simulink model "Battery_SC_NTSMC_NN"  (R2021a)
settings: Solver=ode23tb  StartTime=0.0  StopTime=5  MaxStep=1e-4  RelTol=1e-3
values from neighbouring files (symbols this model uses):
  C = 1e-12    [MPPTNN.m]    (also in NN_Tph.m)
  L = 100e-3    (= 0.1)    [MPPTNN.m]    (also in NN_Tph.m)
  Lf = 10e-3    (= 0.01)    [MPPTNN.m]    (also in NN_Tph.m)
  Ll = 31e-6    (= 3.1e-05)    [MPPTNN.m]    (also in NN_Tph.m)
  R = 4.33    [MPPTNN.m]    (also in NN_Tph.m)
  Rf = 40e-3    (= 0.04)    [MPPTNN.m]    (also in NN_Tph.m)
  RL = 0.1    [MPPTNN.m]    (also in NN_Tph.m)
  Ts = 0.50e-5    (= 5e-06)    [MPPTNN.m]    (also in NN_Tph.m)
undefined symbols (not defined in the file or in its folder): Ion, Lithium, sigbuilder_block
libraries: neural x125, spsFirstOrderFilterLib x11, spsSeriesRLCBranchLib x10, spsIGBTDiodeLib x5, spsPWMGeneratorDCDCLib x5, simulink x5, spsMeanLib x5, pid_lib x4, spsDiodeLib x4, spsabctodq0Lib x3, spsThreePhaseSeriesRLCBranchLib x2, spsRMSLib x2
(part 1 of 4)
settings Model: Creator=Rodayna  LastModifiedBy=Morteza Pirmohammad
settings SolverCC: AlgebraicLoopSolver=TrustRegion
settings DataIOCC: ReturnWorkspaceOutputs=off
settings DebuggingCC: SFMachineParentedDataDiag=warning  ArithmeticOperatorsInVariantConditions=warning
settings SFSimCC: SimUseLocalCustomCode=off  CustomCodeUndefinedFunction=UseInterfaceOnly
settings RTWCC: RTWUseLocalCustomCode=off
settings CodeAppCC: StateflowObjectComments=on
settings SimscapeCC: SimscapeNormalizeSystem=off

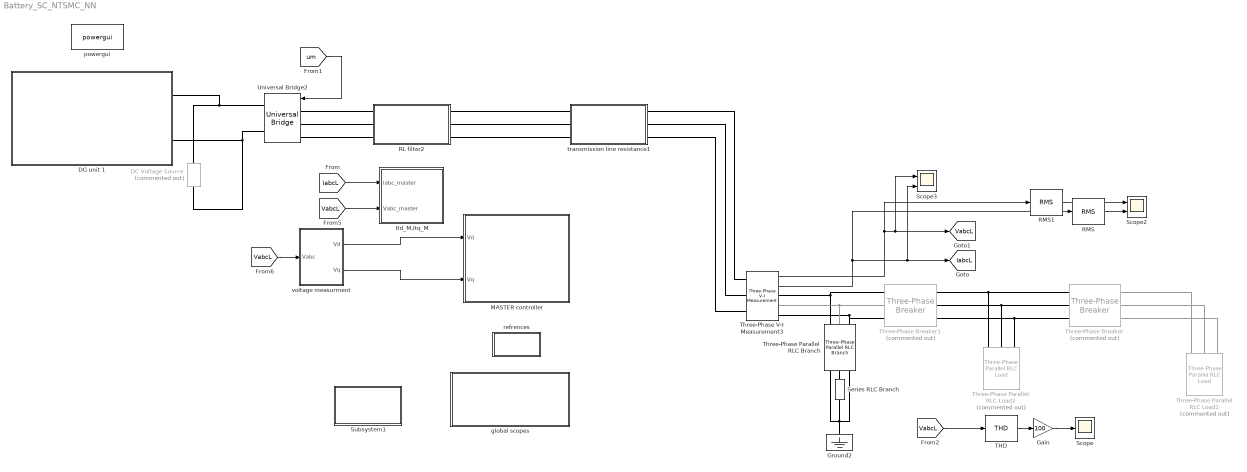
== system Battery_SC_NTSMC_NN ==
  DC Voltage Source : spsDCVoltageSourceLib/DC Voltage Source  Commented=on  Amplitude=100  Measurements=None
  DG unit 1 : Subsystem
  Gain : Gain  Gain=100
  Ground2 : spsGroundLib/Ground  LConnTagsString=a
  Itd_M,Itq_M : Subsystem
  MASTER controller : Subsystem
  RL filter2 : Subsystem
  RMS : spsRMSLib/RMS  TrueRMS=on  Freq=50  RMSInit=0  Ts=0
  RMS1 : spsRMSLib/RMS  TrueRMS=on  Freq=50  RMSInit=0  Ts=0
  Scope : Scope
  Scope2 : Scope  NumInputPorts=2
  Scope3 : Scope  NumInputPorts=2
  Series RLC Branch : spsSeriesRLCBranchLib/Series RLC Branch  LConnTagsString=__new0  RConnTagsString=__new0  BranchType=R  Resistance=0.1  Inductance=1e-3  SetiL0=off  InitialCurrent=0  Capacitance=1e-6  Setx0=off  InitialVoltage=0  Measurements=None
  Subsystem1 : Subsystem
  THD : spsTHDLib/THD  Freq=50  Ts=0
      settings: SourceProductBaseCode=PS
  Three-Phase Parallel RLC Branch : spsThreePhaseParallelRLCBranchLib/Three-Phase Parallel RLC Branch  LConnTagsString=A|B|C  RConnTagsString=A|B|C  BranchType=RLC  Resistance=R  Inductance=L  Capacitance=C  Measurements=Branch voltages and currents
      settings: SourceProductBaseCode=PS
  Three-Phase Parallel RLC Load1 : spsThreePhaseParallelRLCLoadLib/Three-Phase Parallel RLC Load  Commented=on  LConnTagsString=A|B|C  Configuration=Y (grounded)  NominalVoltage=380  Vabc=[1e3 1e3 1e3]  Vabcp=[1e3 1e3 1e3]  NominalFrequency=50  UnbalancedPower=off  ActivePower=5e3  InductivePower=0  CapacitivePower=0  Pabc=[10e3 9e3 11e3]  QLabc=[100 90 110]  QCabc=[100 90 110]  Pabcp=[10e3 9e3 11e3]  QLabcp=[100 90 110]  QCabcp=[100 90 110]  Measurements=None  LoadType=constant Z
  Three-Phase Parallel RLC Load2 : spsThreePhaseParallelRLCLoadLib/Three-Phase Parallel RLC Load  Commented=on  LConnTagsString=A|B|C  Configuration=Y (grounded)  NominalVoltage=380  Vabc=[1e3 1e3 1e3]  Vabcp=[1e3 1e3 1e3]  NominalFrequency=50  UnbalancedPower=off  ActivePower=10e3  InductivePower=5e3  CapacitivePower=0  Pabc=[10e3 9e3 11e3]  QLabc=[100 90 110]  QCabc=[100 90 110]  Pabcp=[10e3 9e3 11e3]  QLabcp=[100 90 110]  QCabcp=[100 90 110]  Measurements=None  LoadType=constant PQ
  Three-Phase V-I Measurement3 : spsThreePhaseVIMeasurementLib/Three-Phase V-I Measurement  VoltageMeasurement=phase-to-ground  SetLabelV=off  LabelV=Vabc  Vpu=off  VpuLL=off  CurrentMeasurement=yes  SetLabelI=off  LabelI=Iabc  Ipu=off  Pbase=100e6  Vbase=500e3  OutputType=Complex  PhasorSimulation=off  PSBequivalent=0
  Three-Phase Breaker : spsThreePhaseBreakerLib/Three-Phase Breaker  Commented=on  InitialState=open  SwitchA=on  SwitchB=on  SwitchC=on  SwitchTimes="[2  3]"  External=off  BreakerResistance=0.01  SnubberResistance=1e6  SnubberCapacitance=inf  Measurements=None
  Three-Phase Breaker1 : spsThreePhaseBreakerLib/Three-Phase Breaker  Commented=on  InitialState=open  SwitchA=on  SwitchB=on  SwitchC=on  SwitchTimes="[1  4]"  External=off  BreakerResistance=0.01  SnubberResistance=1e6  SnubberCapacitance=inf  Measurements=None
  Universal Bridge2 : spsUniversalBridgeLib/Universal Bridge  Arms=3  SnubberResistance=1e3  SnubberCapacitance=inf  Device=MOSFET / Diodes  Ron=1e-3  Lon=0  ForwardVoltages="[  0  0  ]"  ForwardVoltage=0  GTOparameters=[ 10e-6 , 20e-6 ]  IGBTparameters=[ 1e-6 , 2e-6 ]  Measurements=None  Measurements_2=None  converterType=Rectifier
  global scopes : Subsystem
  powergui : spspowerguiLib/powergui  Priority=1  SimulationMode=Discrete  SampleTime=Ts  frequency=60  Iterations=50  frequencyindice=0  Pbase=100e6  ErrMax=1e-4  UnitsV=kV  UnitsW=MW  buscounter=0  FunctionMessages=off  echomessages=off  EnableUseOfTLC=off  CurrentSourceSwitches=off  DisableSnubberDevices=off  DisableRonSwitches=off  DisableVfSwitches=off  DisplayEquations=off  AutomaticDiscreteSolvers=off  SolverType=Tustin/Backward Euler (TBE)  Interpol=off  ExternalGateDelay=off  methode=off  Ts=100  x0status=blocks  SPID=on  SwTol=0  HookPort=off  NonlinearTolerance=1e-4  nMaxIteration=100  ContinueOnMaxIteration=off  RestoreLinks=warning  ResistiveCurrentMeasurement=off  Frange=[0:2:500]  Ylog=off  Xlog=on  ShowGrid=off  save=off  variable=ZData  structure=0  ZoomFFT=off  StartTime=0.0  cycles=1  DisplayStyle=1  fundamental=60  FreqAxis=off  MaxFrequency=1000  frequencyindicesteady=1  RmsSteady=1  display=off
  refrences : Subsystem
  transmission line resistance1 : Subsystem
  voltage measurment : Subsystem
  tag scope: IabcL=global, VabcL=global
  wires:
  voltage measurment/2(Vq) -> MASTER controller/2(Vq)
  voltage measurment/1(Vd) -> MASTER controller/1(Vd)
  [VabcL] -> Itd_M,Itq_M/2(Vabc_master)
  [VabcL] -> voltage measurment/1(Vabc)
  [IabcL] -> Itd_M,Itq_M/1(Iabc_master)
  [um] -> Universal Bridge2/1
  RMS/1 -> Scope2/2
  RMS1/1 -> Scope2/1
  Three-Phase V-I Measurement3/1 -> RMS1/1, Scope3/1, [VabcL]
  Three-Phase V-I Measurement3/2 -> RMS/1, Scope3/2, [IabcL]
  Gain/1 -> Scope/1
  THD/1 -> Gain/1
  [VabcL] -> THD/1
  connections:
  DG unit 1/RConn1 -- Universal Bridge2/RConn1 -- DC Voltage Source/RConn1
  DG unit 1/RConn2 -- DC Voltage Source/LConn1 -- Universal Bridge2/RConn2
  transmission line resistance1/LConn3 -- RL filter2/RConn3
  transmission line resistance1/LConn1 -- RL filter2/RConn1
  RL filter2/RConn2 -- transmission line resistance1/LConn2
  Universal Bridge2/LConn2 -- RL filter2/LConn2
  Universal Bridge2/LConn1 -- RL filter2/LConn1
  Universal Bridge2/LConn3 -- RL filter2/LConn3
  Three-Phase Parallel RLC Branch/LConn3 -- Three-Phase V-I Measurement3/RConn3 -- Three-Phase Breaker1/LConn3
  Three-Phase Parallel RLC Branch/LConn1 -- Three-Phase V-I Measurement3/RConn1 -- Three-Phase Breaker1/LConn1
  Three-Phase Parallel RLC Load2/LConn2 -- Three-Phase Breaker/LConn2 -- Three-Phase Breaker1/RConn2
  Three-Phase Parallel RLC Branch/RConn1 -- Ground2/LConn1 -- Series RLC Branch/RConn1 -- Three-Phase Parallel RLC Branch/RConn3
  Three-Phase Parallel RLC Load2/LConn1 -- Three-Phase Breaker/LConn1 -- Three-Phase Breaker1/RConn1
  Three-Phase Breaker1/LConn2 -- Three-Phase Parallel RLC Branch/LConn2 -- Three-Phase V-I Measurement3/RConn2
  Three-Phase Parallel RLC Load2/LConn3 -- Three-Phase Breaker/LConn3 -- Three-Phase Breaker1/RConn3
  Series RLC Branch/LConn1 -- Three-Phase Parallel RLC Branch/RConn2
  transmission line resistance1/RConn1 -- Three-Phase V-I Measurement3/LConn1
  Three-Phase Breaker/RConn2 -- Three-Phase Parallel RLC Load1/LConn2
  Three-Phase Breaker/RConn3 -- Three-Phase Parallel RLC Load1/LConn3
  Three-Phase V-I Measurement3/LConn2 -- transmission line resistance1/RConn2
  Three-Phase V-I Measurement3/LConn3 -- transmission line resistance1/RConn3
  Three-Phase Breaker/RConn1 -- Three-Phase Parallel RLC Load1/LConn1

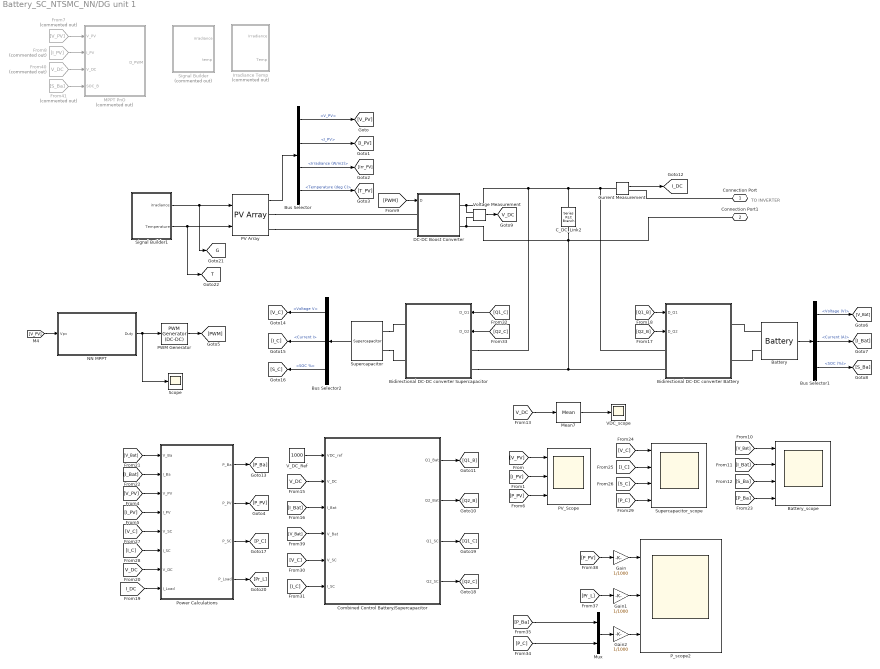
== system Battery_SC_NTSMC_NN/DG unit 1 ==
  note: TO INVERTER
  Battery : spsBatteryLib/Battery  BatType=Lithium-Ion  ShowTempParam=off  ThermalPreset=no  ShowAgeParam=off  NomV=750  NomQ=40  SOC=50  Batt_Tr=0.1  PresetModel=on  MaxQ=40  MinV=562.5  FullV=872.9904  Dis_rate=17.3913  R=0.1875  Normal_OP=36.1739  expZone="[810.2894      1.965217]"  current=[17.5 35 52]  Units=Time  Tci=20  NomT=20  T2=-30  MaxQ2=4.8  FullV2=7.1  Normal_OP2=5.655  expZone2="[6.58           1]"  Rca=0.6  ti=2000  Dp=0  Neq0=0  Tsim=1e6  Ta1=25  Qeol=5.4*0.9  Reol=0.013333*1.2  Char_age=[2.3478, 3]  Dis_age=[2.3478, 10]  N1=1500  N2=10500  N3=1000  N4=1400  Ta2=45  N5=950
  "Battery_scope " : Scope  NumInputPorts=4
  Bidirectional DC-DC converter Battery : Subsystem
  Bidirectional DC-DC converter Supercapacitor : Subsystem
  Bus Selector : BusSelector  OutputSignals=V_PV,I_PV,Irradiance (W/m2),Temperature (deg C)
  Bus Selector1 : BusSelector  OutputSignals=Voltage (V),Current (A),SOC (%)
  Bus Selector2 : BusSelector  OutputSignals=Voltage V,Current I,SOC %
  C_DC_Link2 : spsSeriesRLCBranchLib/Series RLC Branch  LConnTagsString=__new0  RConnTagsString=__new0  BranchType=C  Resistance=1  Inductance=1e-3  SetiL0=off  InitialCurrent=0  Capacitance=500e-6  Setx0=off  InitialVoltage=0  Measurements=None
  Combined Control Battery/Supercapacitor : Subsystem
  Current Measurement : spsCurrentMeasurementLib/Current Measurement  PhasorSimulation=off  OutputType=Complex  PSBequivalent=0
  DC-DC Boost Converter : Subsystem
  From40 : From  Commented=on  GotoTag=V_DC  TagVisibility=global
  From41 : From  Commented=on  GotoTag=S_Ba
  From7 : From  Commented=on  GotoTag=V_PV
  From8 : From  Commented=on  GotoTag=I_PV
  Gain : Gain  Gain=1/1000
  Gain1 : Gain  Gain=1/1000
  Gain2 : Gain  Gain=1/1000
  Irradiance Temp : Subsystem  Tag=STV Subsys  Commented=on  LoadFcn=sigbuilder_block('load');  StartFcn=sigbuilder_block('start');  StopFcn=sigbuilder_block('stop');  ClipboardFcn=sigbuilder_block('clipboard');  mask(Sigbuilder block){tuvar=[0:10]}
      mask help: Sigbuilder GUI
      mask init:
      | if ~strcmp(get_param(bdroot(gcbh),'SimulationStatus'),'stopped') tuvar = sigbuilder_block('maskInit'); end
      settings: CopyFcn=sigbuilder_block('copy');  DeleteFcn=sigbuilder_block('delete');  ModelCloseFcn=sigbuilder_block('modelClose');  PreSaveFcn=sigbuilder_block('preSave');  PauseFcn=sigbuilder_block('pause')  ContinueFcn=sigbuilder_block('continue')  NameChangeFcn=sigbuilder_block('namechange');  OpenFcn=sigbuilder_block('open',[6 0 1012.5 477.75 ]);  CloseFcn=sigbuilder_block('close');
      mask Display: plot(0, 0, 100, 100,[2, 2, 32, 32, 2], [68, 8, 8, 68, 68],[32, 2], [38, 38], [32, 19, 2],[53, 60, 44], [32, 17, 17, 2],[16, 16, 31, 31]);txt = getActiveGroup(gcbh);text(2, 100, txt,'verticalAlignment', 'top');
  MPPT PnO : Subsystem  Commented=on
  Mean7 : spsMeanLib/Mean  Freq=60  Vinit=0  Ts=0
  Mux : Mux  Inputs=2
  NN MPPT : Subsystem
      mask help: Custom Neural Network
      mask Display: e = 0.06;c1 = [120 150 230]/255;c2 = ([120 150 230]+0)/383;c3 = ([120 150 230]+128)/383;patch([0 1 1 0],[0 0 1 1],c1);patch([0 1 1 1-e 1-e 0+e],[0 0 1 1-e 0+e 0+e],c2);patch([0 0 1 1-e 0+e 0+e],[0 1 1 1-e 1-e 0+e],c3);plot([0 1 1 0 0],[0 0 1 1 0]);fprintf('NNET');port_label('input',1,' Input');port_label('output',1,'Output ');
  PV Array : spsPVArrayLib/PV Array  Npar=6  Nser=30  PlotType=array @ 25 deg.C & specified irradiances  S_vec="[ 1000 800 500  250 ]"  Temp_C_vec="[0 25 50  ]"  ModuleName=Yingli Energy (China) YL250P-29b  PlotWhenSelected=on  Pm=250.496  Ncell=60  Voc=38.4  Isc=8.79  Vm=30.4  Im=8.24  beta_Voc_pc=-0.337  alpha_Isc_pc=0.0438  beta_Voc=-0.12941  alpha_Isc=0.00385  IL=8.8005  I0=1.272e-10  nI=0.99849  Rsh=362.5163  Rs=0.42475  RobustModel=off  RobustCellTemperature=313.3991  BAL=on  Tc=Tc  Tfilter=5e-5
  PV_Scope : Scope  NumInputPorts=3
  "PWM Generator " : spsPWMGeneratorDCDCLib/PWM Generator (DC-DC)  Fsw=5000  Ts=0
  P_scope2 : Scope  NumInputPorts=3
  Power Calculations : Subsystem
  Scope : Scope
  Signal Builder : Subsystem  Tag=STV Subsys  Commented=on  LoadFcn=sigbuilder_block('load');  StartFcn=sigbuilder_block('start');  StopFcn=sigbuilder_block('stop');  ClipboardFcn=sigbuilder_block('clipboard');  mask(Sigbuilder block){tuvar=[0:10]}
      mask help: Simulink:masks:SigbuilderBlock_MD
      mask init:
      | if ~strcmp(get_param(bdroot(gcbh),'SimulationStatus'),'stopped') tuvar = sigbuilder_block('maskInit'); end
      settings: CopyFcn=sigbuilder_block('copy');  DeleteFcn=sigbuilder_block('delete');  ModelCloseFcn=sigbuilder_block('modelClose');  PreSaveFcn=sigbuilder_block('preSave');  PauseFcn=sigbuilder_block('pause');  ContinueFcn=sigbuilder_block('continue');  NameChangeFcn=sigbuilder_block('namechange');  OpenFcn=sigbuilder_block('open',[6 0 1012.5 477.75 ]);  CloseFcn=sigbuilder_block('close');
      mask Display: plot(0, 0, 100, 100,[2, 2, 32, 32, 2], [68, 8, 8, 68, 68],[32, 2], [38, 38], [32, 19, 2],[53, 60, 44], [32, 17, 17, 2],[16, 16, 31, 31]);txt = getActiveGroup(gcbh);text(2, 100, txt,'verticalAlignment', 'top');
  Signal Builder1 : Subsystem  Tag=STV Subsys  LoadFcn=sigbuilder_block('load');  StartFcn=sigbuilder_block('start');  StopFcn=sigbuilder_block('stop');  ClipboardFcn=sigbuilder_block('clipboard');  mask(Sigbuilder block){tuvar=[0:10]}
      mask help: Simulink:masks:SigbuilderBlock_MD
      mask init:
      | if ~strcmp(get_param(bdroot(gcbh),'SimulationStatus'),'stopped') tuvar = sigbuilder_block('maskInit'); end
      settings: CopyFcn=sigbuilder_block('copy');  DeleteFcn=sigbuilder_block('delete');  ModelCloseFcn=sigbuilder_block('modelClose');  PreSaveFcn=sigbuilder_block('preSave');  PauseFcn=sigbuilder_block('pause');  ContinueFcn=sigbuilder_block('continue');  NameChangeFcn=sigbuilder_block('namechange');  OpenFcn=sigbuilder_block('open',[0 0 1024.5 518.25 ]);  CloseFcn=sigbuilder_block('close');
      mask Display: plot(0, 0, 100, 100,[2, 2, 32, 32, 2], [68, 8, 8, 68, 68],[32, 2], [38, 38], [32, 19, 2],[53, 60, 44], [32, 17, 17, 2],[16, 16, 31, 31]);txt = getActiveGroup(gcbh);text(2, 100, txt,'verticalAlignment', 'top');
  Supercapacitor : spsSupercapacitorLib/Supercapacitor  C=350  Rdc=0.003  Voltage=820  Ns=1  Np=12  Vinit=820  Temp=25  PresetModel=on  EstParam=off  Nc=1  r=1e-9  epsilon=6.0208e-10  Ich=10  Vstern="[0.161  2.7  7.8]"  Self_dis=on  Ioc=10  Vself="[720  710  701  689]"  demandeplot=off  I="[40 50 100  500]"  Units=sec  Vmax=0  If=0  deltaV=0  alpha=0  sec=0
      settings: SourceProductBaseCode=PS
  Supercapacitor_scope : Scope  NumInputPorts=4
  VDC_scope : Scope
  V_DC_Ref : Constant  Value=1000
  Voltage Measurement : spsVoltageMeasurementLib/Voltage Measurement  PhasorSimulation=off  OutputType=Complex  PSBequivalent=0
  Connection Port : PMIOPort  Side=Right
  Connection Port1 : PMIOPort  Port=2  Side=Right
  tag scope: G=global, I_DC=global, T=global, V_DC=global
  wires:
  [P_C] -> Mux/2
  Bus Selector/2 -> [I_PV]  "<I_PV>"
  [P_PV] -> PV_Scope/3
  Current Measurement/1 -> [I_DC]
  Bus Selector2/1 -> [V_C]  "<Voltage V>"
  [PWM] -> DC-DC Boost Converter/1(D)
  Bus Selector1/2 -> [I_Bat]  "<Current (A)>"
  Bus Selector/4 -> [T_PV]  "<Temperature (deg C)>"
  [I_Bat] -> "Battery_scope "/2
  [V_PV] -> Power Calculations/3(V_PV)
  Power Calculations/4(P_Load) -> [Pr_L]
  [I_PV] -> PV_Scope/2
  Bus Selector1/3 -> [S_Ba]  "<SOC (%)>"
  [Q1_C] -> Bidirectional DC-DC converter Supercapacitor/1(D_Q1)
  Bus Selector2/2 -> [I_C]  "<Current I>"
  Combined Control Battery/Supercapacitor/1(Q1_Bat) -> [Q1_B]
  Combined Control Battery/Supercapacitor/3(Q1_SC) -> [Q1_C]
  From8/1 -> MPPT PnO/2(I_PV)
  [V_C] -> Combined Control Battery/Supercapacitor/5("V_SC ")
  [Q2_C] -> Bidirectional DC-DC converter Supercapacitor/2(D_Q2)
  [S_C] -> Supercapacitor_scope/3
  [S_Ba] -> "Battery_scope "/3
  Battery/1 -> Bus Selector1/1
  Bus Selector1/1 -> [V_Bat]  "<Voltage (V)>"
  Bus Selector/3 -> [Irr_PV]  "<Irradiance (W/m2)>"
  [Q1_B] -> Bidirectional DC-DC converter Battery/1(D_Q1)
  [I_Bat] -> Power Calculations/2(I_Ba)
  Bus Selector/1 -> [V_PV]  "<V_PV>"
  [V_Bat] -> Power Calculations/1(V_Ba)
  [V_DC] -> Power Calculations/7(V_DC)
  [I_C] -> Combined Control Battery/Supercapacitor/6(I_SC)
  [V_Bat] -> Combined Control Battery/Supercapacitor/4(V_Bat)
  Power Calculations/3(P_SC) -> [P_C]
  [V_DC] -> Mean7/1
  Supercapacitor/1 -> Bus Selector2/1
  Power Calculations/2(P_PV) -> [P_PV]
  Bus Selector2/3 -> [S_C]  "<SOC %>"
  From7/1 -> MPPT PnO/1(V_PV)
  PV Array/1 -> Bus Selector/1
  [P_Ba] -> Mux/1
  From40/1 -> MPPT PnO/3(V_DC)
  [V_C] -> Supercapacitor_scope/1
  [I_DC] -> Power Calculations/8(I_Load)
  Combined Control Battery/Supercapacitor/4(Q2_SC) -> [Q2_C]
  [Q2_B] -> Bidirectional DC-DC converter Battery/2(D_Q2)
  Combined Control Battery/Supercapacitor/2(Q2_Bat) -> [Q2_B]
  Mux/1 -> Gain2/1
  Voltage Measurement/1 -> [V_DC]
  From41/1 -> MPPT PnO/4(SOC_B)
  [P_Ba] -> "Battery_scope "/4
  [I_Bat] -> Combined Control Battery/Supercapacitor/3(I_Bat)
  [P_PV] -> Gain/1
  [V_DC] -> Combined Control Battery/Supercapacitor/2(V_DC)
  [P_C] -> Supercapacitor_scope/4
  Mean7/1 -> VDC_scope/1
  [I_PV] -> Power Calculations/4(I_PV)
  [I_C] -> Supercapacitor_scope/2
  [Pr_L] -> Gain1/1
  Power Calculations/1(P_Ba) -> [P_Ba]
  [V_C] -> Power Calculations/5(V_SC)
  [V_Bat] -> "Battery_scope "/1
  [V_PV] -> PV_Scope/1
  [I_C] -> Power Calculations/6(I_SC)
  V_DC_Ref/1 -> Combined Control Battery/Supercapacitor/1(VDC_ref)
  Signal Builder1/2(Temperature) -> PV Array/2, [T]
  Signal Builder1/1(irradiance) -> PV Array/1, [G]
  Gain/1 -> P_scope2/1
  Gain1/1 -> P_scope2/2
  Gain2/1 -> P_scope2/3
  [V_PV] -> NN MPPT/1(Vpv)
  NN MPPT/1(Duty) -> Scope/1, "PWM Generator "/1
  "PWM Generator "/1 -> [PWM]
  connections:
  Bidirectional DC-DC converter Supercapacitor/LConn2 -- Voltage Measurement/LConn2 -- DC-DC Boost Converter/RConn2 -- C_DC_Link2/RConn1 -- Connection Port1/RConn1 -- Bidirectional DC-DC converter Battery/LConn2
  Supercapacitor/LConn1 -- Bidirectional DC-DC converter Supercapacitor/RConn1
  PV Array/RConn1 -- DC-DC Boost Converter/LConn1
  Connection Port/RConn1 -- Current Measurement/RConn1
  PV Array/RConn2 -- DC-DC Boost Converter/LConn2
  Supercapacitor/LConn2 -- Bidirectional DC-DC converter Supercapacitor/RConn2
  Battery/LConn2 -- Bidirectional DC-DC converter Battery/RConn2
  Battery/LConn1 -- Bidirectional DC-DC converter Battery/RConn1
  Current Measurement/LConn1 -- Bidirectional DC-DC converter Battery/LConn1 -- Bidirectional DC-DC converter Supercapacitor/LConn1 -- Voltage Measurement/LConn1 -- DC-DC Boost Converter/RConn1 -- C_DC_Link2/LConn1

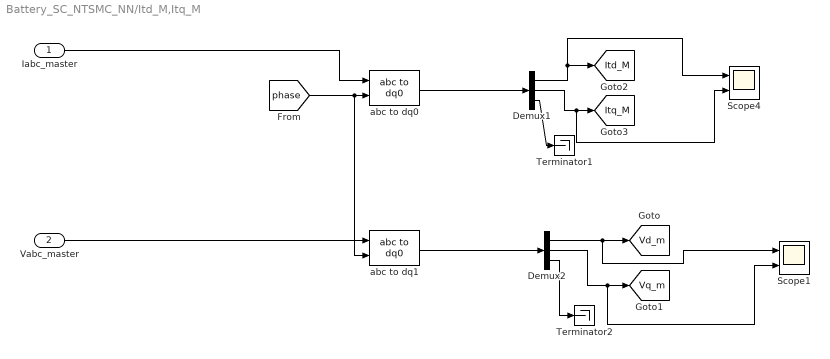
== system Battery_SC_NTSMC_NN/Itd_M,Itq_M ==
  Iabc_master : Inport
  Vabc_master : Inport  Port=2
  Demux1 : Demux  Outputs=3
  Demux2 : Demux  Outputs=3
  Scope1 : Scope  NumInputPorts=2
  Scope4 : Scope  NumInputPorts=2
  Terminator1 : Terminator
  Terminator2 : Terminator
  abc to dq0 : spsabctodq0Lib/abc to dq0  Alignment=90 degrees behind phase A axis
  abc to dq1 : spsabctodq0Lib/abc to dq0  Alignment=90 degrees behind phase A axis
  tag scope: Itd_M=global, Itq_M=global, Vd_m=global, Vq_m=global
  wires:
  Demux1/2 -> Scope4/2, [Itq_M]
  [phase] -> abc to dq1/2, abc to dq0/2
  Demux1/1 -> [Itd_M], Scope4/1
  Demux1/3 -> Terminator1/1
  Iabc_master/1 -> abc to dq0/1
  Demux2/1 -> Scope1/1, [Vd_m]
  Demux2/2 -> Scope1/2, [Vq_m]
  Demux2/3 -> Terminator2/1
  Vabc_master/1 -> abc to dq1/1
  abc to dq0/1 -> Demux1/1
  abc to dq1/1 -> Demux2/1

== system Battery_SC_NTSMC_NN/MASTER controller ==
  Vd : Inport
  Vq : Inport  Port=2
  Demux : Demux  Outputs=3
  NTSMC/NN first layer : Subsystem
  SVPWM Generator (2-Level : spsSVPWMGenerator2LevelLib/SVPWM Generator (2-Level)  InputType=alpha-beta components  SwitchingPattern=Pattern #1  Fc=10000  ParUref=[0.4 0 50]  Ts=0
      settings: SourceProductBaseCode=PS
  Saturation : Saturate  UpperLimit=1  LowerLimit=0  LinearizeAsGain=off  ZeroCross=off
  Scope : Scope  Commented=on
  Scope1 : Scope  Commented=on  NumInputPorts=2
  Scope2 : Scope  Commented=on  NumInputPorts=2
  Terminator : Terminator
  dq0 to Alpha-Beta Zero : spsdq0toAlphaBetaZeroLib/dq0 to Alpha-Beta-Zero  Alignment=90 degrees behind phase A axis
      settings: SourceProductBaseCode=PS
  tag scope: um=global
  wires:
  Demux/3 -> Terminator/1
  [phase] -> dq0 to Alpha-Beta Zero/2
  NTSMC/NN first layer/1(Udq) -> Scope1/2, dq0 to Alpha-Beta Zero/1
  dq0 to Alpha-Beta Zero/1 -> Scope1/1, Demux/1
  SVPWM Generator (2-Level/1 -> Saturation/1
  Demux/1 -> SVPWM Generator (2-Level/1
  Demux/2 -> SVPWM Generator (2-Level/2
  Vd/1 -> Scope2/1, NTSMC/NN first layer/1(Vd)
  Vq/1 -> NTSMC/NN first layer/2(Vq), Scope2/2
  Saturation/1 -> [um], Scope/1

== system Battery_SC_NTSMC_NN/RL filter2 ==
  Three-Phase Series RLC Branch : spsThreePhaseSeriesRLCBranchLib/Three-Phase Series RLC Branch  LConnTagsString=A|B|C  RConnTagsString=A|B|C  BranchType=RL  Resistance=Rf  Inductance=Lf  Capacitance=1e-6  Measurements=None
  Load7 : PMIOPort  Side=Right
  Load8 : PMIOPort  Port=2  Side=Left
  Load9 : PMIOPort  Port=3  Side=Left
  Load10 : PMIOPort  Port=4  Side=Right
  Load11 : PMIOPort  Port=5  Side=Left
  Load12 : PMIOPort  Port=6  Side=Right
  connections:
  Load12/RConn1 -- Three-Phase Series RLC Branch/RConn3
  Load7/RConn1 -- Three-Phase Series RLC Branch/RConn1
  Load10/RConn1 -- Three-Phase Series RLC Branch/RConn2
  Load9/RConn1 -- Three-Phase Series RLC Branch/LConn2
  Load11/RConn1 -- Three-Phase Series RLC Branch/LConn3
  Load8/RConn1 -- Three-Phase Series RLC Branch/LConn1

== system Battery_SC_NTSMC_NN/Subsystem1 ==
  MATLAB Function : MATLAB Function  TreatAsAtomicUnit=on
  MATLAB Function1 : MATLAB Function  TreatAsAtomicUnit=on
  tag scope: P_L=global, Q_L=global
  wires:
  [Vd_m] -> MATLAB Function/2(Vd), MATLAB Function1/2(Vd)
  MATLAB Function1/1(QL) -> [Q_L]
  MATLAB Function/1(pL) -> [P_L]
  [Itq_M] -> MATLAB Function1/1(ILq)
  [Itd_M] -> MATLAB Function/1(ILd)

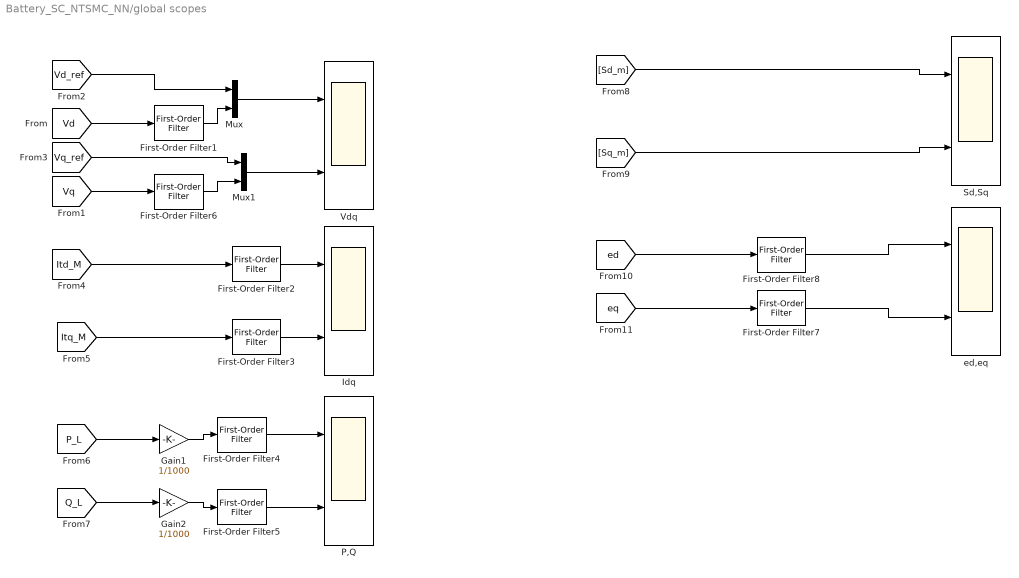
== system Battery_SC_NTSMC_NN/global scopes ==
  First-Order Filter{1..8} (8 alike) : spsFirstOrderFilterLib/First-Order Filter  FilterType=Lowpass  Tc=10e-3  Ts=0  Initialize=off  Vac_Init=[0, 0, 60]  Vdc_Init=0  PlotResponse=off  FreqRange="[0,  200,  1]"
  Gain1 : Gain  Gain=1/1000
  Gain2 : Gain  Gain=1/1000
  Idq : Scope  NumInputPorts=2
  Mux : Mux  Inputs=2
  Mux1 : Mux  Inputs=2
  P,Q : Scope  NumInputPorts=2
  Sd,Sq : Scope  NumInputPorts=2
  Vdq : Scope  NumInputPorts=2
  ed,eq : Scope  NumInputPorts=2
  wires:
  [Vd_ref] -> Mux/1
  [Vd] -> First-Order Filter1/1
  [Vq_ref] -> Mux1/1
  [Vq] -> First-Order Filter6/1
  [Itd_M] -> First-Order Filter2/1
  [Itq_M] -> First-Order Filter3/1
  [P_L] -> Gain1/1
  [Q_L] -> Gain2/1
  Mux/1 -> Vdq/1
  Mux1/1 -> Vdq/2
  First-Order Filter2/1 -> Idq/1
  First-Order Filter3/1 -> Idq/2
  First-Order Filter4/1 -> P,Q/1
  First-Order Filter5/1 -> P,Q/2
  First-Order Filter1/1 -> Mux/2
  First-Order Filter6/1 -> Mux1/2
  Gain1/1 -> First-Order Filter4/1
  Gain2/1 -> First-Order Filter5/1
  [Sd_m] -> Sd,Sq/1
  [Sq_m] -> Sd,Sq/2
  First-Order Filter8/1 -> ed,eq/1
  First-Order Filter7/1 -> ed,eq/2
  [ed] -> First-Order Filter8/1
  [eq] -> First-Order Filter7/1

== system Battery_SC_NTSMC_NN/refrences ==
  Constant1 : Constant  Value=311.1  LockScale=on
  Constant2 : Constant  Value=0  LockScale=on
  Discrete Virtual PLL : Subsystem  DialogController=POWERSYS.PowerSysDialog  mask(Discrete Virtual PLL){Freq=50, Phase=0, Ts=Ts}
      mask prompts: Freq "Frequency (Hz):"; Phase "Phase (degrees):"; Ts "Sample time:"
      mask help:
      | This virtual PLL has no input signal. The block simulates the outputs of an actual PLL by  using the parameters specified in the mask.
      |
      | Output 1: Frequency (Hz)
      | Output 2: Vectorized output  [sin(wt)  cos(wt)]
      | Output 3: wt in rad/s (varying from 0 to 2*pi)
      mask init:
      | power_initmask();
      mask Display: disp('')
  Scope3 : Scope
  Terminator1 : Terminator
  Terminator2 : Terminator
  tag scope: Vd_ref=global, Vq_ref=global, phase=global
  wires:
  Constant1/1 -> [Vd_ref]
  Constant2/1 -> [Vq_ref]
  Discrete Virtual PLL/1(Freq) -> Terminator1/1
  Discrete Virtual PLL/2(Sin_Cos) -> Terminator2/1
  Discrete Virtual PLL/3(wt) -> [phase], Scope3/1

== system Battery_SC_NTSMC_NN/transmission line resistance1 ==
  Three-Phase Series RLC Branch : spsThreePhaseSeriesRLCBranchLib/Three-Phase Series RLC Branch  LConnTagsString=A|B|C  RConnTagsString=A|B|C  BranchType=RL  Resistance=RL  Inductance=Ll  Capacitance=1e-6  Measurements=None
  Load7 : PMIOPort  Side=Right
  Load8 : PMIOPort  Port=2  Side=Left
  Load9 : PMIOPort  Port=3  Side=Left
  Load10 : PMIOPort  Port=4  Side=Right
  Load11 : PMIOPort  Port=5  Side=Left
  Load12 : PMIOPort  Port=6  Side=Right
  connections:
  Three-Phase Series RLC Branch/LConn2 -- Load9/RConn1
  Three-Phase Series RLC Branch/LConn1 -- Load8/RConn1
  Three-Phase Series RLC Branch/LConn3 -- Load11/RConn1
  Load7/RConn1 -- Three-Phase Series RLC Branch/RConn1
  Three-Phase Series RLC Branch/RConn2 -- Load10/RConn1
  Load12/RConn1 -- Three-Phase Series RLC Branch/RConn3

== system Battery_SC_NTSMC_NN/voltage measurment ==
  Vabc : Inport
  Demux : Demux  Outputs=3
  Terminator : Terminator
  abc to dq0 : spsabctodq0Lib/abc to dq0  Alignment=90 degrees behind phase A axis
  Vd : Outport
  Vq : Outport  Port=2
  tag scope: Vd=global, Vq=global
  wires:
  Vabc/1 -> abc to dq0/1
  [phase] -> abc to dq0/2
  Demux/2 -> [Vq], Vq/1
  Demux/1 -> Vd/1, [Vd]
  Demux/3 -> Terminator/1
  abc to dq0/1 -> Demux/1

== system Battery_SC_NTSMC_NN/DG unit 1/Bidirectional DC-DC converter Battery ==
  D_Q1 : Inport
  D_Q2 : Inport  Port=2
  L_Bidirectional : spsSeriesRLCBranchLib/Series RLC Branch  LConnTagsString=__new0  RConnTagsString=__new0  BranchType=RL  Resistance=0.05  Inductance=0.3e-3  SetiL0=off  InitialCurrent=0  Capacitance=1e-6  Setx0=off  InitialVoltage=0  Measurements=None
  Q1 : spsIGBTDiodeLib/IGBT//Diode  Ron=1e-3  Rs=1e5  Cs=inf  Measurements=on
  Q2 : spsIGBTDiodeLib/IGBT//Diode  Ron=1e-3  Rs=1e5  Cs=inf  Measurements=on
  Terminator : Terminator
  Terminator1 : Terminator
  High + : PMIOPort  Side=Left
  Low + : PMIOPort  Port=2  Side=Right
  High - : PMIOPort  Port=3  Side=Left
  Low - : PMIOPort  Port=4  Side=Right
  wires:
  D_Q2/1 -> Q2/1
  D_Q1/1 -> Q1/1
  Q1/1 -> Terminator/1
  Q2/1 -> Terminator1/1
  connections:
  High -/RConn1 -- Low -/RConn1 -- Q2/RConn1
  High +/RConn1 -- Q1/LConn1
  Low +/RConn1 -- L_Bidirectional/RConn1
  Q2/LConn1 -- L_Bidirectional/LConn1 -- Q1/RConn1

== system Battery_SC_NTSMC_NN/DG unit 1/Bidirectional DC-DC converter Supercapacitor ==
  D_Q1 : Inport
  D_Q2 : Inport  Port=2
  L_Bidirectional : spsSeriesRLCBranchLib/Series RLC Branch  LConnTagsString=__new0  RConnTagsString=__new0  BranchType=RL  Resistance=0.05  Inductance=0.355e-3  SetiL0=off  InitialCurrent=0  Capacitance=1e-6  Setx0=off  InitialVoltage=0  Measurements=None
  L_Boost1 : spsSeriesRLCBranchLib/Series RLC Branch  LConnTagsString=__new0  RConnTagsString=__new0  BranchType=L  Resistance=0.05  Inductance=1.5e-3  SetiL0=off  InitialCurrent=0  Capacitance=1e-6  Setx0=off  InitialVoltage=0  Measurements=None
  Q1 : spsIGBTDiodeLib/IGBT//Diode  Ron=1e-3  Rs=1e5  Cs=inf  Measurements=on
  Q2 : spsIGBTDiodeLib/IGBT//Diode  Ron=1e-3  Rs=1e5  Cs=inf  Measurements=on
  Terminator : Terminator
  Terminator1 : Terminator
  High + : PMIOPort  Side=Left
  Low + : PMIOPort  Port=2  Side=Right
  High - : PMIOPort  Port=3  Side=Left
  Low - : PMIOPort  Port=4  Side=Right
  wires:
  D_Q2/1 -> Q2/1
  D_Q1/1 -> Q1/1
  Q1/1 -> Terminator/1
  Q2/1 -> Terminator1/1
  connections:
  High -/RConn1 -- Low -/RConn1 -- Q2/RConn1
  Low +/RConn1 -- L_Bidirectional/RConn1
  Q2/LConn1 -- L_Bidirectional/LConn1 -- Q1/RConn1
  L_Boost1/RConn1 -- Q1/LConn1
  L_Boost1/LConn1 -- High +/RConn1

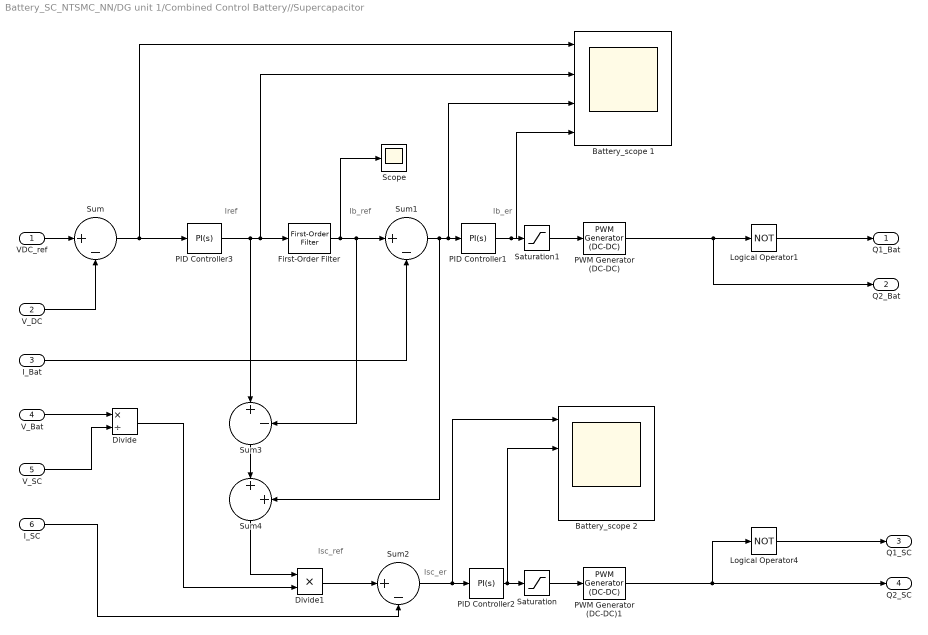
== system Battery_SC_NTSMC_NN/DG unit 1/Combined Control Battery//Supercapacitor ==
  note: Iref
  note: Ib_ref
  note: Ib_er
  note: Isc_ref
  note: Isc_er
  VDC_ref : Inport
  V_DC : Inport  Port=2
  I_Bat : Inport  Port=3
  V_Bat : Inport  Port=4
  "V_SC " : Inport  Port=5
  I_SC : Inport  Port=6
  Battery_scope 1 : Scope  NumInputPorts=4
  Battery_scope 2 : Scope  NumInputPorts=4
  Divide : Product  Inputs=*/
  Divide1 : Product  Inputs=**
  First-Order Filter : spsFirstOrderFilterLib/First-Order Filter  FilterType=Lowpass  Tc=0.015  Ts=0  Initialize=off  Vac_Init=[0, 0, 60]  Vdc_Init=0  PlotResponse=off  FreqRange="[0,  200,  1]"
  Logical Operator1 : Logic  Operator=NOT  AllPortsSameDT=off  OutDataTypeStr=boolean
  Logical Operator4 : Logic  Operator=NOT  AllPortsSameDT=off  OutDataTypeStr=boolean
  PID Controller1 : pid_lib/PID Controller  Controller=PI  Form=Parallel  TimeDomain=Continuous-time  UseExternalTs=off  SampleTime=-1  IntegratorMethod=Forward Euler  FilterMethod=Forward Euler  ControllerParametersSource=internal  P=0.03  I=0.5  D=0  UseFilter=on  N=100  TunerSelectOption=Transfer Function Based (PID Tuner App)  InitialConditionSource=internal  InitialConditionForIntegrator=0  InitialConditionForFilter=0  DifferentiatorICPrevScaledInput=0  ExternalReset=none  TrackingMode=off  Kt=1  LimitOutput=off  SatLimitsSource=internal  UpperSaturationLimit=inf  LowerSaturationLimit=-inf  LinearizeAsGain=on  AntiWindupMode=none  Kb=1  POutMin=[]  POutMax=[]  IOutMin=[]  IOutMax=[]  DOutMin=[]  DOutMax=[]  NOutMin=[]  NOutMax=[]  SumOutMin=[]  SumOutMax=[]  SaturationOutMin=[]  SaturationOutMax=[]  PParamMin=[]  PParamMax=[]  IParamMin=[]  IParamMax=[]  DParamMin=[]  DParamMax=[]  NParamMin=[]  NParamMax=[]  KbParamMin=[]  KbParamMax=[]  KtParamMin=[]  KtParamMax=[]  KbOutMin=[]  KbOutMax=[]  KtOutMin=[]  KtOutMax=[]  IntegratorOutMin=[]  IntegratorOutMax=[]  FilterOutMin=[]  FilterOutMax=[]  SumI1OutMin=[]  SumI1OutMax=[]  SumI2OutMin=[]  SumI2OutMax=[]  SumI3OutMin=[]  SumI3OutMax=[]  SumI4OutMin=[]  SumI4OutMax=[]  SumDOutMin=[]  SumDOutMax=[]  DifferentiatorOutMin=[]  DifferentiatorOutMax=[]  FilterDiffOutCoefMin=[]  FilterDiffOutCoefMax=[]  ReciprocalOutMin=[]  ReciprocalOutMax=[]  SumDenOutMin=[]  SumDenOutMax=[]  SumNumOutMin=[]  SumNumOutMax=[]  DivideOutMin=[]  DivideOutMax=[]  UdiffTsProdOutMin=[]  UdiffTsProdOutMax=[]  NTsProdOutMin=[]  NTsProdOutMax=[]  UintegralTsProdOutMin=[]  UintegralTsProdOutMax=[]  UngainTsProdOutMin=[]  UngainTsProdOutMax=[]  IntegratorContinuousStateAttributes=''  IntegratorStateMustResolveToSignalObject=off  IntegratorRTWStateStorageClass=Auto  FilterContinuousStateAttributes=''  FilterStateMustResolveToSignalObject=off  FilterRTWStateStorageClass=Auto  ParallelPVariant=InternalParameters  IdealPVariant=Disabled  IVariant=InternalParameters  DVariant=Disabled  IntegratorVariant=Continuous  SatVariant=Disabled  AWVariant=Passthrough  PCopyVariant=Disabled  TRVariant=Disabled  FdbkBlocksVariant=Forward  IdealPFdbkVariant=Disabled  SatFdbkVariant=Disabled  DerivativeFilterVariant=Disabled  NVariant=Disabled  NCopyVariant=Disabled_SignalSpec  FilterICVariant=Disabled  IntegratorICVariant=InternalICs  ExternalResetVariant=Disabled  TRSumVariant=Passthrough  SumFdbkVariant=Disabled  SumVariant=Sum_PI  TsampFilterVariant=InternalTs  TsampNgainVariant=Passthrough  TsampIntegralVariant=Passthrough  ExternalSaturationOutDataTypeStr=Inherit: Same as second input
  PID Controller2 : pid_lib/PID Controller  Controller=PI  Form=Parallel  TimeDomain=Continuous-time  UseExternalTs=off  SampleTime=-1  IntegratorMethod=Forward Euler  FilterMethod=Forward Euler  ControllerParametersSource=internal  P=0.75  I=100  D=0  UseFilter=on  N=100  TunerSelectOption=Transfer Function Based (PID Tuner App)  InitialConditionSource=internal  InitialConditionForIntegrator=0  InitialConditionForFilter=0  DifferentiatorICPrevScaledInput=0  ExternalReset=none  TrackingMode=off  Kt=1  LimitOutput=off  SatLimitsSource=internal  UpperSaturationLimit=inf  LowerSaturationLimit=-inf  LinearizeAsGain=on  AntiWindupMode=none  Kb=1  POutMin=[]  POutMax=[]  IOutMin=[]  IOutMax=[]  DOutMin=[]  DOutMax=[]  NOutMin=[]  NOutMax=[]  SumOutMin=[]  SumOutMax=[]  SaturationOutMin=[]  SaturationOutMax=[]  PParamMin=[]  PParamMax=[]  IParamMin=[]  IParamMax=[]  DParamMin=[]  DParamMax=[]  NParamMin=[]  NParamMax=[]  KbParamMin=[]  KbParamMax=[]  KtParamMin=[]  KtParamMax=[]  KbOutMin=[]  KbOutMax=[]  KtOutMin=[]  KtOutMax=[]  IntegratorOutMin=[]  IntegratorOutMax=[]  FilterOutMin=[]  FilterOutMax=[]  SumI1OutMin=[]  SumI1OutMax=[]  SumI2OutMin=[]  SumI2OutMax=[]  SumI3OutMin=[]  SumI3OutMax=[]  SumI4OutMin=[]  SumI4OutMax=[]  SumDOutMin=[]  SumDOutMax=[]  DifferentiatorOutMin=[]  DifferentiatorOutMax=[]  FilterDiffOutCoefMin=[]  FilterDiffOutCoefMax=[]  ReciprocalOutMin=[]  ReciprocalOutMax=[]  SumDenOutMin=[]  SumDenOutMax=[]  SumNumOutMin=[]  SumNumOutMax=[]  DivideOutMin=[]  DivideOutMax=[]  UdiffTsProdOutMin=[]  UdiffTsProdOutMax=[]  NTsProdOutMin=[]  NTsProdOutMax=[]  UintegralTsProdOutMin=[]  UintegralTsProdOutMax=[]  UngainTsProdOutMin=[]  UngainTsProdOutMax=[]  IntegratorContinuousStateAttributes=''  IntegratorStateMustResolveToSignalObject=off  IntegratorRTWStateStorageClass=Auto  FilterContinuousStateAttributes=''  FilterStateMustResolveToSignalObject=off  FilterRTWStateStorageClass=Auto  ParallelPVariant=InternalParameters  IdealPVariant=Disabled  IVariant=InternalParameters  DVariant=Disabled  IntegratorVariant=Continuous  SatVariant=Disabled  AWVariant=Passthrough  PCopyVariant=Disabled  TRVariant=Disabled  FdbkBlocksVariant=Forward  IdealPFdbkVariant=Disabled  SatFdbkVariant=Disabled  DerivativeFilterVariant=Disabled  NVariant=Disabled  NCopyVariant=Disabled_SignalSpec  FilterICVariant=Disabled  IntegratorICVariant=InternalICs  ExternalResetVariant=Disabled  TRSumVariant=Passthrough  SumFdbkVariant=Disabled  SumVariant=Sum_PI  TsampFilterVariant=InternalTs  TsampNgainVariant=Passthrough  TsampIntegralVariant=Passthrough  ExternalSaturationOutDataTypeStr=Inherit: Same as second input
  PID Controller3 : pid_lib/PID Controller  Controller=PI  Form=Parallel  TimeDomain=Continuous-time  UseExternalTs=off  SampleTime=-1  IntegratorMethod=Forward Euler  FilterMethod=Forward Euler  ControllerParametersSource=internal  P=1.4  I=100  D=0  UseFilter=on  N=100  TunerSelectOption=Transfer Function Based (PID Tuner App)  InitialConditionSource=internal  InitialConditionForIntegrator=0  InitialConditionForFilter=0  DifferentiatorICPrevScaledInput=0  ExternalReset=none  TrackingMode=off  Kt=1  LimitOutput=off  SatLimitsSource=internal  UpperSaturationLimit=inf  LowerSaturationLimit=-inf  LinearizeAsGain=on  AntiWindupMode=none  Kb=1  POutMin=[]  POutMax=[]  IOutMin=[]  IOutMax=[]  DOutMin=[]  DOutMax=[]  NOutMin=[]  NOutMax=[]  SumOutMin=[]  SumOutMax=[]  SaturationOutMin=[]  SaturationOutMax=[]  PParamMin=[]  PParamMax=[]  IParamMin=[]  IParamMax=[]  DParamMin=[]  DParamMax=[]  NParamMin=[]  NParamMax=[]  KbParamMin=[]  KbParamMax=[]  KtParamMin=[]  KtParamMax=[]  KbOutMin=[]  KbOutMax=[]  KtOutMin=[]  KtOutMax=[]  IntegratorOutMin=[]  IntegratorOutMax=[]  FilterOutMin=[]  FilterOutMax=[]  SumI1OutMin=[]  SumI1OutMax=[]  SumI2OutMin=[]  SumI2OutMax=[]  SumI3OutMin=[]  SumI3OutMax=[]  SumI4OutMin=[]  SumI4OutMax=[]  SumDOutMin=[]  SumDOutMax=[]  DifferentiatorOutMin=[]  DifferentiatorOutMax=[]  FilterDiffOutCoefMin=[]  FilterDiffOutCoefMax=[]  ReciprocalOutMin=[]  ReciprocalOutMax=[]  SumDenOutMin=[]  SumDenOutMax=[]  SumNumOutMin=[]  SumNumOutMax=[]  DivideOutMin=[]  DivideOutMax=[]  UdiffTsProdOutMin=[]  UdiffTsProdOutMax=[]  NTsProdOutMin=[]  NTsProdOutMax=[]  UintegralTsProdOutMin=[]  UintegralTsProdOutMax=[]  UngainTsProdOutMin=[]  UngainTsProdOutMax=[]  IntegratorContinuousStateAttributes=''  IntegratorStateMustResolveToSignalObject=off  IntegratorRTWStateStorageClass=Auto  FilterContinuousStateAttributes=''  FilterStateMustResolveToSignalObject=off  FilterRTWStateStorageClass=Auto  ParallelPVariant=InternalParameters  IdealPVariant=Disabled  IVariant=InternalParameters  DVariant=Disabled  IntegratorVariant=Continuous  SatVariant=Disabled  AWVariant=Passthrough  PCopyVariant=Disabled  TRVariant=Disabled  FdbkBlocksVariant=Forward  IdealPFdbkVariant=Disabled  SatFdbkVariant=Disabled  DerivativeFilterVariant=Disabled  NVariant=Disabled  NCopyVariant=Disabled_SignalSpec  FilterICVariant=Disabled  IntegratorICVariant=InternalICs  ExternalResetVariant=Disabled  TRSumVariant=Passthrough  SumFdbkVariant=Disabled  SumVariant=Sum_PI  TsampFilterVariant=InternalTs  TsampNgainVariant=Passthrough  TsampIntegralVariant=Passthrough  ExternalSaturationOutDataTypeStr=Inherit: Same as second input
  PWM Generator (DC-DC) : spsPWMGeneratorDCDCLib/PWM Generator (DC-DC)  Fsw=16000  Ts=0
  PWM Generator (DC-DC)1 : spsPWMGeneratorDCDCLib/PWM Generator (DC-DC)  Fsw=16000  Ts=0
  Saturation : Saturate  UpperLimit=1  LowerLimit=0
  Saturation1 : Saturate  UpperLimit=1  LowerLimit=0
  Scope : Scope
  Sum{,1..3} (4 alike) : Sum  Inputs=|+-
  Sum4 : Sum  Inputs=|++
  Q1_Bat : Outport
  Q2_Bat : Outport  Port=2
  Q1_SC : Outport  Port=3
  Q2_SC : Outport  Port=4
  wires:
  First-Order Filter/1 -> Sum3/2, Sum1/1, Scope/1
  Saturation1/1 -> PWM Generator (DC-DC)/1
  PID Controller1/1 -> Saturation1/1, Battery_scope 1/4
  Saturation/1 -> PWM Generator (DC-DC)1/1
  PID Controller2/1 -> Saturation/1, Battery_scope 2/2
  Sum4/1 -> Divide1/1
  Divide/1 -> Divide1/2
  Divide1/1 -> Sum2/1
  Sum3/1 -> Sum4/1
  PID Controller3/1 -> Sum3/1, First-Order Filter/1, Battery_scope 1/2
  PWM Generator (DC-DC)1/1 -> Logical Operator4/1, Q2_SC/1
  Logical Operator4/1 -> Q1_SC/1
  "V_SC "/1 -> Divide/2
  V_Bat/1 -> Divide/1
  V_DC/1 -> Sum/2
  VDC_ref/1 -> Sum/1
  Sum/1 -> PID Controller3/1, Battery_scope 1/1
  Logical Operator1/1 -> Q1_Bat/1
  Sum2/1 -> PID Controller2/1, Battery_scope 2/1
  I_SC/1 -> Sum2/2
  I_Bat/1 -> Sum1/2
  PWM Generator (DC-DC)/1 -> Q2_Bat/1, Logical Operator1/1
  Sum1/1 -> Sum4/2, PID Controller1/1, Battery_scope 1/3

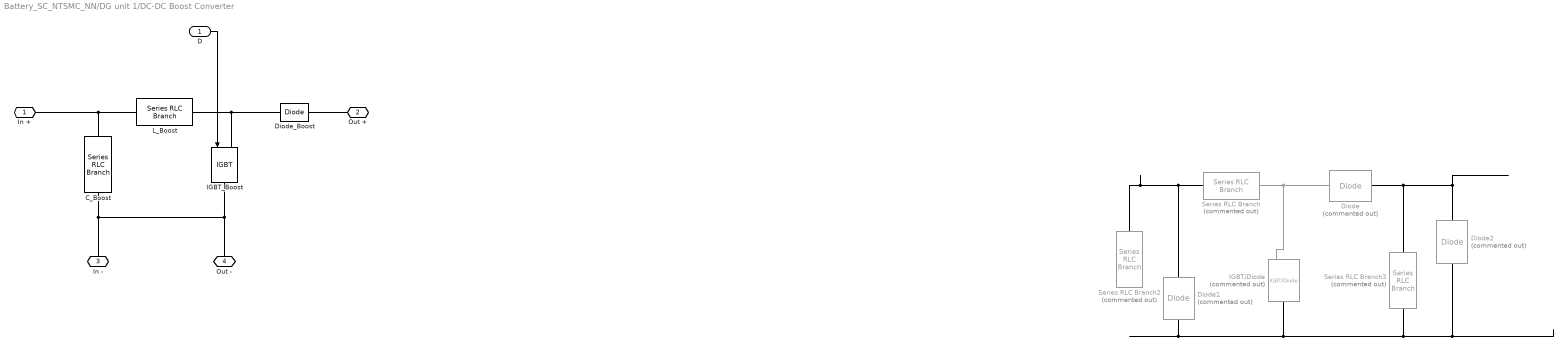
== system Battery_SC_NTSMC_NN/DG unit 1/DC-DC Boost Converter ==
  D : Inport
  C_Boost : spsSeriesRLCBranchLib/Series RLC Branch  LConnTagsString=__new0  RConnTagsString=__new0  BranchType=C  Resistance=0.01  Inductance=1e-3  SetiL0=off  InitialCurrent=0  Capacitance=2200e-6  Setx0=off  InitialVoltage=0  Measurements=None
  Diode : spsDiodeLib/Diode  Commented=on  Ron=0.5  Lon=0  Vf=0.7  IC=0  UseSnubber=0  Rs=1e5  Cs=250e-9  Measurements=off
  Diode1 : spsDiodeLib/Diode  Commented=on  Ron=0.5  Lon=0  Vf=0.7  IC=0  UseSnubber=0  Rs=1e5  Cs=250e-9  Measurements=off
  Diode2 : spsDiodeLib/Diode  Commented=on  Ron=0.5  Lon=0  Vf=0.7  IC=0  UseSnubber=0  Rs=1e5  Cs=250e-9  Measurements=off
  Diode_Boost : spsDiodeLib/Diode  Ron=1e-4  Lon=0  Vf=0  IC=0  UseSnubber=off  Rs=inf  Cs=inf  Measurements=off
  IGBT/Diode : spsIGBTDiodeLib/IGBT//Diode  Commented=on  Ron=1e-4  Rs=1e5  Cs=inf  Measurements=off
  IGBT_Boost : spsIGBTLib/IGBT  Ron=0.001  Lon=0  Vf=0  Tf=0  Tt=0  IC=0  Rs=1e5  Cs=inf  Measurements=off
  L_Boost : spsSeriesRLCBranchLib/Series RLC Branch  LConnTagsString=__new0  RConnTagsString=__new0  BranchType=RL  Resistance=0.05  Inductance=0.352e-3  SetiL0=off  InitialCurrent=0  Capacitance=1e-6  Setx0=off  InitialVoltage=0  Measurements=None
  Series RLC Branch : spsSeriesRLCBranchLib/Series RLC Branch  Commented=on  LConnTagsString=__new0  RConnTagsString=__new0  BranchType=L  Resistance=0.001  Inductance=0.7e-1  SetiL0=off  InitialCurrent=0  Capacitance=1e-6  Setx0=off  InitialVoltage=0  Measurements=None
  Series RLC Branch2 : spsSeriesRLCBranchLib/Series RLC Branch  Commented=on  LConnTagsString=__new0  RConnTagsString=__new0  BranchType=C  Resistance=6  Inductance=1e-3  SetiL0=off  InitialCurrent=0  Capacitance=470e-6  Setx0=off  InitialVoltage=0  Measurements=None
  Series RLC Branch3 : spsSeriesRLCBranchLib/Series RLC Branch  Commented=on  LConnTagsString=__new0  RConnTagsString=__new0  BranchType=C  Resistance=6  Inductance=1e-3  SetiL0=off  InitialCurrent=0  Capacitance=1000e-6  Setx0=off  InitialVoltage=0  Measurements=None
  In + : PMIOPort  Side=Left
  Out + : PMIOPort  Port=2  Side=Right
  In - : PMIOPort  Port=3  Side=Left
  Out - : PMIOPort  Port=4  Side=Right
  wires:
  D/1 -> IGBT_Boost/1
  ? -> IGBT/Diode/1
  connections:
  In +/RConn1 -- C_Boost/LConn1 -- L_Boost/LConn1
  L_Boost/RConn1 -- IGBT_Boost/LConn1 -- Diode_Boost/LConn1
  IGBT/Diode/RConn1 -- Diode2/LConn1 -- Series RLC Branch3/RConn1 -- Diode1/LConn1
  Series RLC Branch/LConn1 -- Diode1/RConn1 -- Series RLC Branch2/LConn1
  IGBT/Diode/LConn1 -- Diode/LConn1 -- Series RLC Branch/RConn1
  Diode/RConn1 -- Series RLC Branch3/LConn1 -- Diode2/RConn1
  Out +/RConn1 -- Diode_Boost/RConn1
  IGBT_Boost/RConn1 -- C_Boost/RConn1 -- In -/RConn1 -- Out -/RConn1

== system Battery_SC_NTSMC_NN/DG unit 1/Irradiance Temp ==
  Demux : Demux  Tag=STV Demux  Outputs=2
      settings: DisplayOption=none
  FromWs : FromWorkspace  Tag=STV FromWs  VariableName=tuvar
      SigBuilderData=|
      | common.afterFinalStr = 'Extrapolate'
      | common.sampleTime = '0'
      | dataSet.timeRange = [0 2]
      | dataSet.name = 'Constant Irradiance'
      | sbobj.Groups.Name = 'Constant Irradiance'
      | sbobj.Groups.Signals(1).Name = 'Irradiance'
      | sbobj.Groups.Signals(1).XData = [0 0.5 0.5 1.5 1.5 2]
      | sbobj.Groups.Signals(1).YData = [1000 1000 500 500 1000 1000]
      | sbobj.Groups.Signals(2).Name = 'Temp'
      | sbobj.Groups.Signals(2).XData = [0 0.8 0.8 2]
      | sbobj.Groups.Signals(2).YData = [25 25 23 23]
      | sbobj.Groups.TimeRange = [0 2]
  Irradiance : Outport  Tag=STV Outport
  Temp : Outport  Tag=STV Outport  Port=2
  wires:
  FromWs/1 -> Demux/1
  Demux/1 -> Irradiance/1
  Demux/2 -> Temp/1

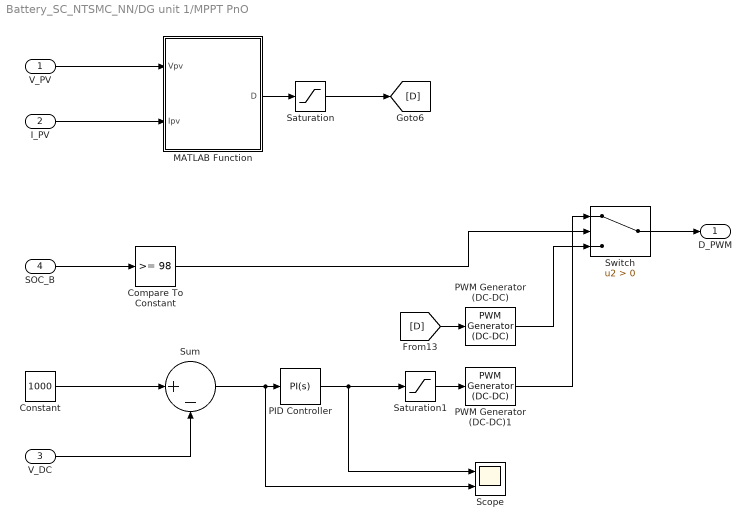
== system Battery_SC_NTSMC_NN/DG unit 1/MPPT PnO ==
  V_PV : Inport
  I_PV : Inport  Port=2
  V_DC : Inport  Port=3
  SOC_B : Inport  Port=4
  Compare To Constant : simulink/Logic and Bit Operations/Compare To Constant  relop=>=  const=98  OutDataTypeStr=boolean
  Constant : Constant  Value=1000
  MATLAB Function : MATLAB Function  TreatAsAtomicUnit=on
  PID Controller : pid_lib/PID Controller  Controller=PI  Form=Parallel  TimeDomain=Continuous-time  UseExternalTs=off  SampleTime=-1  IntegratorMethod=Forward Euler  FilterMethod=Forward Euler  ControllerParametersSource=internal  P=0.5  I=0.5  D=0  UseFilter=on  N=100  TunerSelectOption=Transfer Function Based (PID Tuner App)  InitialConditionSource=internal  InitialConditionForIntegrator=0  InitialConditionForFilter=0  DifferentiatorICPrevScaledInput=0  ExternalReset=none  TrackingMode=off  Kt=1  LimitOutput=off  SatLimitsSource=internal  UpperSaturationLimit=inf  LowerSaturationLimit=-inf  LinearizeAsGain=on  AntiWindupMode=none  Kb=1  POutMin=[]  POutMax=[]  IOutMin=[]  IOutMax=[]  DOutMin=[]  DOutMax=[]  NOutMin=[]  NOutMax=[]  SumOutMin=[]  SumOutMax=[]  SaturationOutMin=[]  SaturationOutMax=[]  PParamMin=[]  PParamMax=[]  IParamMin=[]  IParamMax=[]  DParamMin=[]  DParamMax=[]  NParamMin=[]  NParamMax=[]  KbParamMin=[]  KbParamMax=[]  KtParamMin=[]  KtParamMax=[]  KbOutMin=[]  KbOutMax=[]  KtOutMin=[]  KtOutMax=[]  IntegratorOutMin=[]  IntegratorOutMax=[]  FilterOutMin=[]  FilterOutMax=[]  SumI1OutMin=[]  SumI1OutMax=[]  SumI2OutMin=[]  SumI2OutMax=[]  SumI3OutMin=[]  SumI3OutMax=[]  SumI4OutMin=[]  SumI4OutMax=[]  SumDOutMin=[]  SumDOutMax=[]  DifferentiatorOutMin=[]  DifferentiatorOutMax=[]  FilterDiffOutCoefMin=[]  FilterDiffOutCoefMax=[]  ReciprocalOutMin=[]  ReciprocalOutMax=[]  SumDenOutMin=[]  SumDenOutMax=[]  SumNumOutMin=[]  SumNumOutMax=[]  DivideOutMin=[]  DivideOutMax=[]  UdiffTsProdOutMin=[]  UdiffTsProdOutMax=[]  NTsProdOutMin=[]  NTsProdOutMax=[]  UintegralTsProdOutMin=[]  UintegralTsProdOutMax=[]  UngainTsProdOutMin=[]  UngainTsProdOutMax=[]  IntegratorContinuousStateAttributes=''  IntegratorStateMustResolveToSignalObject=off  IntegratorRTWStateStorageClass=Auto  FilterContinuousStateAttributes=''  FilterStateMustResolveToSignalObject=off  FilterRTWStateStorageClass=Auto  ParallelPVariant=InternalParameters  IdealPVariant=Disabled  IVariant=InternalParameters  DVariant=Disabled  IntegratorVariant=Continuous  SatVariant=Disabled  AWVariant=Passthrough  PCopyVariant=Disabled  TRVariant=Disabled  FdbkBlocksVariant=Forward  IdealPFdbkVariant=Disabled  SatFdbkVariant=Disabled  DerivativeFilterVariant=Disabled  NVariant=Disabled  NCopyVariant=Disabled_SignalSpec  FilterICVariant=Disabled  IntegratorICVariant=InternalICs  ExternalResetVariant=Disabled  TRSumVariant=Passthrough  SumFdbkVariant=Disabled  SumVariant=Sum_PI  TsampFilterVariant=InternalTs  TsampNgainVariant=Passthrough  TsampIntegralVariant=Passthrough  ExternalSaturationOutDataTypeStr=Inherit: Same as second input
  PWM Generator (DC-DC) : spsPWMGeneratorDCDCLib/PWM Generator (DC-DC)  Fsw=5000  Ts=0
  PWM Generator (DC-DC)1 : spsPWMGeneratorDCDCLib/PWM Generator (DC-DC)  Fsw=5000  Ts=0
  Saturation : Saturate
  Saturation1 : Saturate
  Scope : Scope  NumInputPorts=2
  Sum : Sum  Inputs=|+-
  Switch : Switch  Criteria=u2 > Threshold
  D_PWM : Outport
  wires:
  Saturation/1 -> [D]
  [D] -> PWM Generator (DC-DC)/1
  I_PV/1 -> MATLAB Function/2(Ipv)
  V_PV/1 -> MATLAB Function/1(Vpv)
  MATLAB Function/1(D) -> Saturation/1
  Sum/1 -> Scope/2, PID Controller/1
  V_DC/1 -> Sum/2
  Constant/1 -> Sum/1
  PID Controller/1 -> Scope/1, Saturation1/1
  Switch/1 -> D_PWM/1
  Saturation1/1 -> PWM Generator (DC-DC)1/1
  Compare To Constant/1 -> Switch/2
  SOC_B/1 -> Compare To Constant/1
  PWM Generator (DC-DC)/1 -> Switch/3
  PWM Generator (DC-DC)1/1 -> Switch/1

== system Battery_SC_NTSMC_NN/DG unit 1/NN MPPT ==
  note: vmp
  Vpv : Inport
  Constant : Constant  Value=1000
  Mux : Mux  Inputs=2
  NN controller : Subsystem
      mask help: Function Fitting Neural Network
      mask Display: e = 0.06;c1 = [120 150 230]/255;c2 = ([120 150 230]+0)/383;c3 = ([120 150 230]+128)/383;patch([0 1 1 0],[0 0 1 1],c1);patch([0 1 1 1-e 1-e 0+e],[0 0 1 1-e 0+e 0+e],c2);patch([0 0 1 1-e 0+e 0+e],[0 1 1 1-e 1-e 0+e],c3);plot([0 1 1 0 0],[0 0 1 1 0]);fprintf('NNET');port_label('input',1,' Input');port_label('output',1,'Output ');
  Reshape : Reshape
  Scope : Scope
  Duty : Outport
  wires:
  Mux/1 -> Reshape/1
  Vpv/1 -> Mux/1
  Reshape/1 -> NN controller/1(Input)
  Constant/1 -> Mux/2
  NN controller/1(Output) -> Scope/1, Duty/1

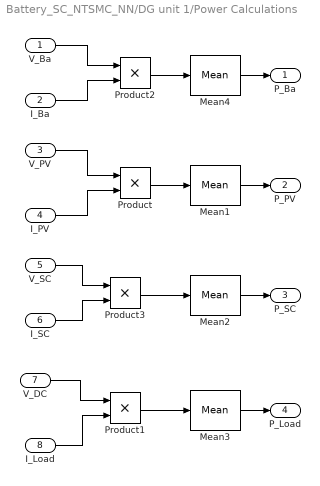
== system Battery_SC_NTSMC_NN/DG unit 1/Power Calculations ==
  V_Ba : Inport
  I_Ba : Inport  Port=2
  V_PV : Inport  Port=3
  I_PV : Inport  Port=4
  V_SC : Inport  Port=5
  I_SC : Inport  Port=6
  V_DC : Inport  Port=7
  I_Load : Inport  Port=8
  Mean{1..4} (4 alike) : spsMeanLib/Mean  Freq=60  Vinit=0  Ts=0
  Product{,1..3} (4 alike) : Product
  P_Ba : Outport
  P_PV : Outport  Port=2
  P_SC : Outport  Port=3
  P_Load : Outport  Port=4
  wires:
  I_Ba/1 -> Product2/2
  V_Ba/1 -> Product2/1
  V_PV/1 -> Product/1
  I_PV/1 -> Product/2
  V_DC/1 -> Product1/1
  I_Load/1 -> Product1/2
  V_SC/1 -> Product3/1
  I_SC/1 -> Product3/2
  Mean4/1 -> P_Ba/1
  Product2/1 -> Mean4/1
  Mean1/1 -> P_PV/1
  Product/1 -> Mean1/1
  Mean2/1 -> P_SC/1
  Product3/1 -> Mean2/1
  Mean3/1 -> P_Load/1
  Product1/1 -> Mean3/1

== system Battery_SC_NTSMC_NN/DG unit 1/Signal Builder ==
  Demux : Demux  Tag=STV Demux  Outputs=2
      settings: DisplayOption=none
  FromWs : FromWorkspace  Tag=STV FromWs  VariableName=tuvar
      SigBuilderData=|
      | common.afterFinalStr = 'Extrapolate'
      | common.sampleTime = 0
      | dataSet.timeRange = [0 10]
      | dataSet.name = 'Group 1'
      | sbobj.Groups.Name = 'Group 1'
      | sbobj.Groups.Signals(1).Name = 'irradiance'
      | sbobj.Groups.Signals(1).XData = [0 0.5 0.5 1.5 1.5 10]
      | sbobj.Groups.Signals(1).YData = [1000 1000 500 500 1000 1000]
      | sbobj.Groups.Signals(2).Name = 'temp'
      | sbobj.Groups.Signals(2).XData = [0 0.8 0.8 10]
      | sbobj.Groups.Signals(2).YData = [25 25 23 23]
  irradiance : Outport  Tag=STV Outport
  temp : Outport  Tag=STV Outport  Port=2
  wires:
  FromWs/1 -> Demux/1
  Demux/1 -> irradiance/1
  Demux/2 -> temp/1

== system Battery_SC_NTSMC_NN/DG unit 1/Signal Builder1 ==
  Demux : Demux  Tag=STV Demux  Outputs=2
      settings: DisplayOption=none
  FromWs : FromWorkspace  Tag=STV FromWs  VariableName=tuvar
      SigBuilderData=|
      | common.afterFinalStr = 'Extrapolate'
      | common.sampleTime = 0
      | dataSet.timeRange = [0 5]
      | dataSet.name = 'Group 1'
      | sbobj.Groups.Name = 'Group 1'
      | sbobj.Groups.Signals(1).Name = 'irradiance'
      | sbobj.Groups.Signals(1).XData = [0 1.505 3.5 5]
      | sbobj.Groups.Signals(1).YData = [1000 995 500 1000]
      | sbobj.Groups.Signals(2).Name = 'Temperature'
      | sbobj.Groups.Signals(2).XData = [0 3.7 5]
      | sbobj.Groups.Signals(2).YData = [24.8 24.64 24.46]
      | sbobj.Groups.TimeRange = [0 5]
  irradiance : Outport  Tag=STV Outport
  Temperature : Outport  Tag=STV Outport  Port=2
  wires:
  FromWs/1 -> Demux/1
  Demux/1 -> irradiance/1
  Demux/2 -> Temperature/1

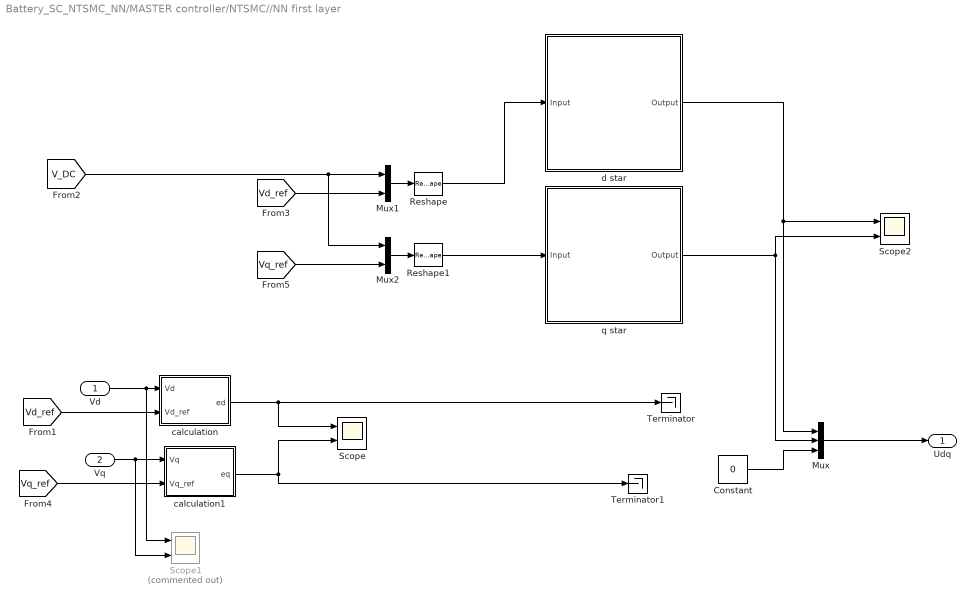
== system Battery_SC_NTSMC_NN/MASTER controller/NTSMC//NN first layer ==
  Vd : Inport
  Vq : Inport  Port=2
  Constant : Constant  Value=0  OutDataTypeStr=double
  Mux : Mux  Inputs=3
  Mux1 : Mux  Inputs=2
  Mux2 : Mux  Inputs=2
  Reshape : Reshape
  Reshape1 : Reshape
  Scope : Scope  NumInputPorts=2
  Scope1 : Scope  Commented=on  NumInputPorts=2
  Scope2 : Scope  NumInputPorts=2
  Terminator : Terminator
  Terminator1 : Terminator
  calculation : Subsystem
  calculation1 : Subsystem
  d star : Subsystem
      mask help: Function Fitting Neural Network
      mask Display: e = 0.06;c1 = [120 150 230]/255;c2 = ([120 150 230]+0)/383;c3 = ([120 150 230]+128)/383;patch([0 1 1 0],[0 0 1 1],c1);patch([0 1 1 1-e 1-e 0+e],[0 0 1 1-e 0+e 0+e],c2);patch([0 0 1 1-e 0+e 0+e],[0 1 1 1-e 1-e 0+e],c3);plot([0 1 1 0 0],[0 0 1 1 0]);fprintf('NNET');port_label('input',1,' Input');port_label('output',1,'Output ');
  q star : Subsystem
      mask help: Function Fitting Neural Network
      mask Display: e = 0.06;c1 = [120 150 230]/255;c2 = ([120 150 230]+0)/383;c3 = ([120 150 230]+128)/383;patch([0 1 1 0],[0 0 1 1],c1);patch([0 1 1 1-e 1-e 0+e],[0 0 1 1-e 0+e 0+e],c2);patch([0 0 1 1-e 0+e 0+e],[0 1 1 1-e 1-e 0+e],c3);plot([0 1 1 0 0],[0 0 1 1 0]);fprintf('NNET');port_label('input',1,' Input');port_label('output',1,'Output ');
  Udq : Outport
  wires:
  calculation1/1(eq) -> Terminator1/1, Scope/2
  Constant/1 -> Mux/3
  Vd/1 -> Scope1/1, calculation/1(Vd)
  Vq/1 -> Scope1/2, calculation1/1(Vq)
  Mux/1 -> Udq/1
  [Vq_ref] -> calculation1/2(Vq_ref)
  [Vd_ref] -> calculation/2(Vd_ref)
  Mux1/1 -> Reshape/1
  Reshape/1 -> d star/1(Input)
  Mux2/1 -> Reshape1/1
  Reshape1/1 -> q star/1(Input)
  calculation/1(ed) -> Terminator/1, Scope/1
  [Vd_ref] -> Mux1/2
  [Vq_ref] -> Mux2/2
  [V_DC] -> Mux2/1, Mux1/1
  d star/1(Output) -> Mux/1, Scope2/1
  q star/1(Output) -> Scope2/2, Mux/2
